simulink model "ForceField_and_Reaching_Phantom"  (R2023b)
settings: Solver=VariableStepAuto  StartTime=0.0  StopTime=10.0  RelTol=1e-3
libraries: PhanTorque_3Dof_Library_64Bits x2, simulink x1, vrlib x1
settings Model: Creator=terri  LastModifiedBy=terri

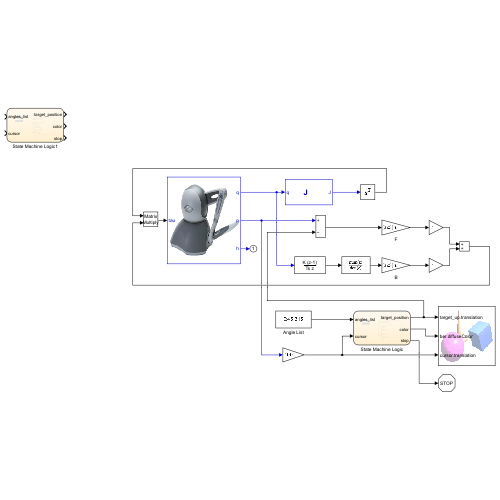
[thumbnail: Simulink's stored preview of the top-level diagram]
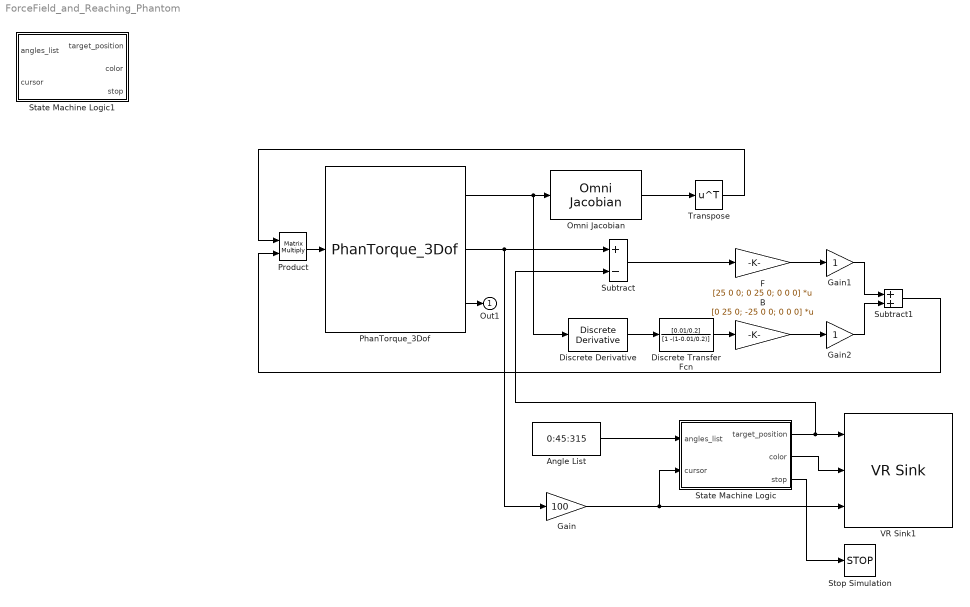
== system ForceField_and_Reaching_Phantom ==
  Angle List : Constant  Value=0:45:315
  B : Gain  Gain=[0 25 0; -25 0 0; 0 0 0]  Multiplication=Matrix(K*u)
  Discrete Derivative : simulink/Discrete/Discrete Derivative  gainval=1.0  ICPrevScaledInput=0.0  OutMin=[]  OutMax=[]  OutDataType=fixdt(1, 16)  OutScaling=2^-10  DoSatur=off
  Discrete Transfer Fcn : DiscreteTransferFcn  Numerator=[0.01/0.2]  Denominator=[1 -(1-0.01/0.2)]
  F : Gain  Gain=[25 0 0; 0 25 0; 0 0 0]  Multiplication=Matrix(K*u)
  Gain : Gain  Gain=100
  Gain1 : Gain
  Gain2 : Gain
  Omni Jacobian : PhanTorque_3Dof_Library_64Bits/Omni Jacobian  SystemSampleTime=-1  VariantActivationTime=update diagram  AllowFlexibleInterface=on  Latency=0  AutoFrameSizeCalculation=off
  PhanTorque_3Dof : PhanTorque_3Dof_Library_64Bits/PhanTorque_3Dof  Haptic_Name='Default Device'
  Product : Product  Multiplication=Matrix(*)
  State Machine Logic : Stateflow chart  TreatAsAtomicUnit=on
      settings: PortSchema="{\"entries\":[{\"content\":{\"sides\":[{\"content\":{\"connectorIds\":[\"In1\",\"In2\"]},\"type\":\"ConnectorPlacement.EquallySpacedRectSide\",\"uuid\":\"2012c964-2602-4c80-977b-ac7ca7ae8f5b\"},{\"content\":{\"connectorIds\":[\"Out2\",\"Out1\",\"Out3\"],\"side\":\"RIGHT\"},\"type\":\"ConnectorPlacement.EquallySpacedRectSide\",\"uuid\":\"01c6fc3b-ba25-4dd7-b95f-3fc66d6fa31c\"},{\"content\":{\"side\":\"TOP\"},\"type\":\"ConnectorPlacement.EquallySpacedRectSide\",\"uuid\":\"0e349c8b-fff0-4cce-a38e-56f1937a9eb7\"}]},\"type\":\"ConnectorPlacement.EquallySpacedConnector\",\"uuid\":\"0aec7ed3-d29a-41fc-b2f0-597bb4555e1d\"}],\"packageUris\":[\"http://schema.mathworks.com/mf0/Connector/R2020b\"],\"version\":\"1.0\"}"
  State Machine Logic1 : Stateflow chart  TreatAsAtomicUnit=on
      settings: PortSchema="{\"entries\":[{\"content\":{\"sides\":[{\"content\":{\"connectorIds\":[\"In1\",\"In2\"]},\"type\":\"ConnectorPlacement.EquallySpacedRectSide\",\"uuid\":\"2012c964-2602-4c80-977b-ac7ca7ae8f5b\"},{\"content\":{\"connectorIds\":[\"Out2\",\"Out1\",\"Out3\"],\"side\":\"RIGHT\"},\"type\":\"ConnectorPlacement.EquallySpacedRectSide\",\"uuid\":\"01c6fc3b-ba25-4dd7-b95f-3fc66d6fa31c\"},{\"content\":{\"side\":\"TOP\"},\"type\":\"ConnectorPlacement.EquallySpacedRectSide\",\"uuid\":\"0e349c8b-fff0-4cce-a38e-56f1937a9eb7\"}]},\"type\":\"ConnectorPlacement.EquallySpacedConnector\",\"uuid\":\"0aec7ed3-d29a-41fc-b2f0-597bb4555e1d\"}],\"packageUris\":[\"http://schema.mathworks.com/mf0/Connector/R2020b\"],\"version\":\"1.0\"}"
  Stop Simulation : Stop
  Subtract : Sum  Inputs=+-
  Subtract1 : Sum
  Transpose : Math  Operator=transpose
  VR Sink1 : vrlib/VR Sink  InstantiateOnLoad=on  SampleTime=0.01  ViewEnable=on  RemoteChange=off  RemoteView=off  FieldsWritten=target_up.translation.3.1.1.double#ber.diffuseColor.3.1.1.double#cursor.translation.3.1.1.double  WorldFileName=2_palline_color.wrl  AutoView=off  VideoDimensions=[]  AllowVariableSize=off
  Out1 : Outport
  wires:
  Gain2/1 -> Subtract1/2
  Product/1 -> PhanTorque_3Dof/1
  Gain1/1 -> Subtract1/1
  Transpose/1 -> Product/1
  Subtract1/1 -> Product/2
  Discrete Transfer Fcn/1 -> B/1
  PhanTorque_3Dof/2 -> Subtract/1, Gain/1
  PhanTorque_3Dof/1 -> Discrete Derivative/1, Omni Jacobian/1
  F/1 -> Gain1/1
  PhanTorque_3Dof/3 -> Out1/1
  Subtract/1 -> F/1
  Discrete Derivative/1 -> Discrete Transfer Fcn/1
  Omni Jacobian/1 -> Transpose/1
  State Machine Logic/1(color) -> VR Sink1/2
  State Machine Logic/2(target_position) -> VR Sink1/1, Subtract/2
  State Machine Logic/3(stop) -> Stop Simulation/1
  Angle List/1 -> State Machine Logic/1(angles_list)
  Gain/1 -> State Machine Logic/2(cursor), VR Sink1/3
  B/1 -> Gain2/1

== stateflow chart ForceField_and_Reaching_Phantom/State Machine Logic ==
  state Start
    entry:
    index = 1;
  state RandomAngleGeneration
    entry:
    random_angles_list = randomAngle(angles_list);
    idx = 1;
  state ShowTarget
    entry:
    color = [1 0.2 0.2];
    target_position = computeTargetPose(random_angles_list(idx));
  state ReachingTargetColor
    entry:
    color = [0 0.8 1];
  state HomeTarget
    entry:
    target_position = [0 0 0];
    color = [1 0.2 0.2];
  state HomeTargetColor
    entry:
    color = [0 0.5 0];
  state Finish
    stop = 1;
  (default) -> Start [order 1]
  (default) -> Start [order 2]
  Start -> RandomAngleGeneration
  (junction 73) -> RandomAngleGeneration
  (junction 72) -> (junction 73)
  RandomAngleGeneration -> ShowTarget
  (junction 78) -> ShowTarget : after(2, sec)[sqrt((target_position(1)-cursor(1))^2 + (target_position(2)-cursor(2))^2) <= 0.2 & i < 2 & idx ~= 8]{idx = idx + 1}
  ShowTarget -> ReachingTargetColor : [sqrt((target_position(1)-cursor(1))^2 + (target_position(2)-cursor(2))^2) <= 0.2 & idx <= 8]
  ReachingTargetColor -> ShowTarget [order 1] : [sqrt((target_position(1)-cursor(1))^2 + (target_position(2)-cursor(2))^2) > 0.2 ]
  ReachingTargetColor -> HomeTarget [order 2] : after(1, sec)[sqrt((target_position(1)-cursor(1))^2 + (target_position(2)-cursor(2))^2) <= 0.2]
  HomeTarget -> HomeTargetColor : [sqrt((target_position(1)-cursor(1))^2 + (target_position(2)-cursor(2))^2) <= 0.2]
  HomeTargetColor -> HomeTarget [order 1] : [sqrt((target_position(1)-cursor(1))^2 + (target_position(2)-cursor(2))^2) > 0.2]
  HomeTargetColor -> (junction 78) [order 4]
  HomeTargetColor -> Finish [order 2] : [idx == 2 & index == 2]
  HomeTargetColor -> (junction 76) [order 3]
  (junction 76) -> (junction 72) : after(2, sec)[idx == 8 & sqrt((target_position(1)-cursor(1))^2 + (target_position(2)-cursor(2))^2) < 0.2 ]{index = index+1}
  data: list_of_angle function_input; random_list function_output; angle function_input; coordinates function_output; angles_list input; color output; cursor input; target_position output; idx local; random_angles_list local; index local; stop output =0
  function random_list = randomAngle(list_of_angle):
    | function random_list = randomAngle(list_of_angle)
    |     size_list = length(list_of_angle);
    |     
    |     % To compute a new seed at each call
    |     rng('shuffle');
    |     % Compute a new permutation at each call using the seed
    |     random_index = randperm(size_list);
    |     
    |     % Initialize the new list with the lenght of al
    |     new_list = zeros(size_list, 1);
    | 
    |     for i = 1:size_list
    |         % Assign the element of al in random order
    |         new_list(i) = list_of_angle(random_index(i));
    |     end
    | 
    |     random_list = new_list;
    | end
  function coordinates = computeTargetPose(angle):
    | function coordinates = computeTargetPose(angle)
    |     % Convert from degrees to radiants
    |     theta = deg2rad(angle);
    | 
    |     % Compute the point's coordinates on the circle
    |     x = 10 * cos(theta);
    |     y = 10 * sin(theta);
    |     z = 0;
    |     coordinates = [x y z];
    | end

== stateflow chart ForceField_and_Reaching_Phantom/State Machine Logic1 ==
  state Start
    entry:
    index = 1;
  state RandomAngleGeneration
    entry:
    random_angles_list = randomAngle(angles_list);
    idx = 1;
  state ShowTarget
    entry:
    color = [1 0.2 0.2];
    target_position = computeTargetPose(random_angles_list(idx));
  state ReachingTargetColor
    entry:
    color = [0 0.8 1];
  state HomeTarget
    entry:
    target_position = [0 0 0];
    color = [1 0.2 0.2];
  state HomeTargetColor
    entry:
    color = [0 0.5 0];
  state Finish
    stop = 1;
  (default) -> Start [order 1]
  (default) -> Start [order 2]
  Start -> RandomAngleGeneration
  (junction 73) -> RandomAngleGeneration
  (junction 72) -> (junction 73)
  RandomAngleGeneration -> ShowTarget
  (junction 78) -> ShowTarget : after(2, sec)[sqrt((target_position(1)-cursor(1))^2 + (target_position(2)-cursor(2))^2) <= 0.2 & i < 2 & idx ~= 8]{idx = idx + 1}
  ShowTarget -> ReachingTargetColor : [sqrt((target_position(1)-cursor(1))^2 + (target_position(2)-cursor(2))^2) <= 0.2 & idx <= 8]
  ReachingTargetColor -> ShowTarget [order 1] : [sqrt((target_position(1)-cursor(1))^2 + (target_position(2)-cursor(2))^2) > 0.2 ]
  ReachingTargetColor -> HomeTarget [order 2] : after(1, sec)[sqrt((target_position(1)-cursor(1))^2 + (target_position(2)-cursor(2))^2) <= 0.2]
  HomeTarget -> HomeTargetColor : [sqrt((target_position(1)-cursor(1))^2 + (target_position(2)-cursor(2))^2) <= 0.2]
  HomeTargetColor -> HomeTarget [order 1] : [sqrt((target_position(1)-cursor(1))^2 + (target_position(2)-cursor(2))^2) > 0.2]
  HomeTargetColor -> (junction 78) [order 4]
  HomeTargetColor -> Finish [order 2] : [idx == 2 & index == 2]
  HomeTargetColor -> (junction 76) [order 3]
  (junction 76) -> (junction 72) : after(2, sec)[idx == 8 & sqrt((target_position(1)-cursor(1))^2 + (target_position(2)-cursor(2))^2) < 0.2 ]{index = index+1}
  data: list_of_angle function_input; random_list function_output; angle function_input; coordinates function_output; angles_list input; color output; cursor input; target_position output; idx local; random_angles_list local; index local; stop output =0
  function random_list = randomAngle(list_of_angle):
    | function random_list = randomAngle(list_of_angle)
    |     size_list = length(list_of_angle);
    |     
    |     % To compute a new seed at each call
    |     rng('shuffle');
    |     % Compute a new permutation at each call using the seed
    |     random_index = randperm(size_list);
    |     
    |     % Initialize the new list with the lenght of al
    |     new_list = zeros(size_list, 1);
    | 
    |     for i = 1:size_list
    |         % Assign the element of al in random order
    |         new_list(i) = list_of_angle(random_index(i));
    |     end
    | 
    |     random_list = new_list;
    | end
  function coordinates = computeTargetPose(angle):
    | function coordinates = computeTargetPose(angle)
    |     % Convert from degrees to radiants
    |     theta = deg2rad(angle);
    | 
    |     % Compute the point's coordinates on the circle
    |     x = 10 * cos(theta);
    |     y = 10 * sin(theta);
    |     z = 0;
    |     coordinates = [x y z];
    | end
